simulink model "trail2"  (R2014a)
settings: Solver=ode45  StartTime=0.0  StopTime=10.0  RelTol=1e-3
libraries: simulink x1
settings Model: Creator=Mostafa  LastModifiedBy=Mostafa

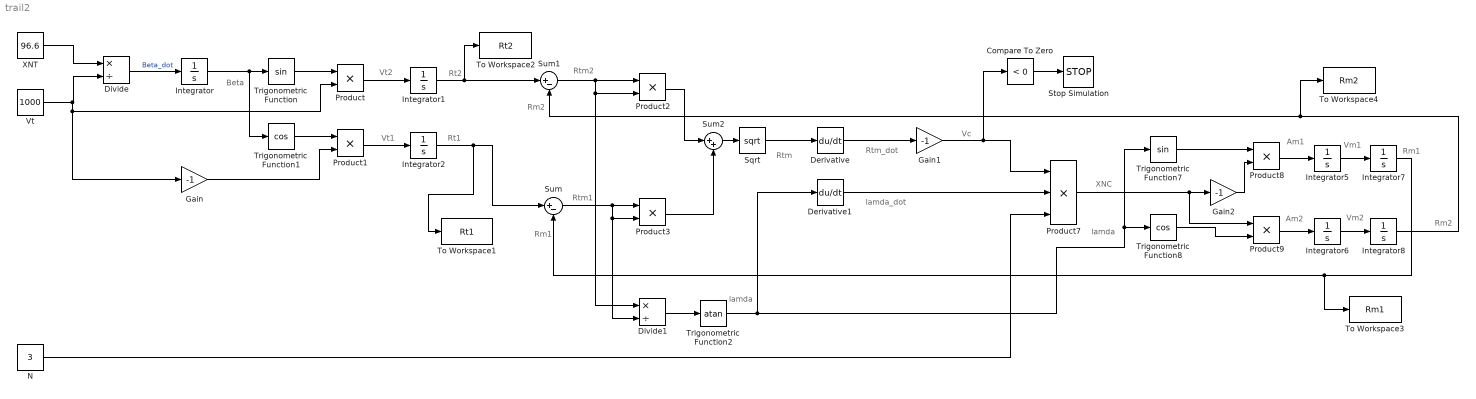
== system trail2 ==
  note: Rm2
  note: Rm1
  note: Vm1
  note: Vm2
  note: Am2
  note: Am1
  note: lamda
  note: XNC
  note: lamda_dot
  note: Vc
  note: Rtm_dot
  note: Rtm
  note: lamda
  note: Rtm2
  note: Rm2
  note: Rtm1
  note: Rm1
  note: Rt1
  note: Rt2
  note: Vt2
  note: Vt1
  note: Beta
  Compare To Zero : simulink/Logic and Bit Operations/Compare To Zero  relop=<  OutDataTypeStr=boolean  ZeroCross=off
  Derivative : Derivative
  Derivative1 : Derivative
  Divide : Product  Inputs=*/
  Divide1 : Product  Inputs=*/
  Gain : Gain  Gain=-1
  Gain1 : Gain  Gain=-1
  Gain2 : Gain  Gain=-1
  Integrator{,5..7} (4 alike) : Integrator
  Integrator1 : Integrator  InitialCondition=10000
  Integrator2 : Integrator  InitialCondition=12000
  Integrator8 : Integrator  InitialCondition=9000
  N : Constant  Value=3
  Product{,1..3,8..9} (6 alike) : Product
  Product7 : Product  Inputs=3
  Sqrt : Sqrt  SaturateOnIntegerOverflow=on
  Stop Simulation : Stop
  Sum : Sum  Inputs=|+-
  Sum1 : Sum  Inputs=|+-
  Sum2 : Sum  Inputs=|++
  To Workspace1 : ToWorkspace  VariableName=Rt1  SampleTime=-1
  To Workspace2 : ToWorkspace  VariableName=Rt2  SampleTime=-1
  To Workspace3 : ToWorkspace  VariableName=Rm1  SampleTime=-1
  To Workspace4 : ToWorkspace  VariableName=Rm2  SampleTime=-1
  Trigonometric Function : Trigonometry
  Trigonometric Function1 : Trigonometry  Operator=cos
  Trigonometric Function2 : Trigonometry  Operator=atan
  Trigonometric Function7 : Trigonometry
  Trigonometric Function8 : Trigonometry  Operator=cos
  "Vt " : Constant  Value=1000
  XNT : Constant  Value=96.6
  wires:
  XNT/1 -> Divide/1
  "Vt "/1 -> Gain/1, Product/2, Divide/2
  Divide/1 -> Integrator/1  "Beta_dot"
  Integrator/1 -> Trigonometric Function1/1, Trigonometric Function/1
  Trigonometric Function/1 -> Product/1
  Gain/1 -> Product1/2
  Trigonometric Function1/1 -> Product1/1
  Product1/1 -> Integrator2/1
  Product/1 -> Integrator1/1
  Integrator1/1 -> To Workspace2/1, Sum1/1
  Integrator2/1 -> To Workspace1/1, Sum/1
  Sum1/1 -> Product2/2, Divide1/1, Product2/1
  Sum/1 -> Divide1/2, Product3/2, Product3/1
  Product2/1 -> Sum2/1
  Product3/1 -> Sum2/2
  Sum2/1 -> Sqrt/1
  Divide1/1 -> Trigonometric Function2/1
  Trigonometric Function2/1 -> Derivative1/1, Trigonometric Function7/1, Trigonometric Function8/1
  Sqrt/1 -> Derivative/1
  Derivative/1 -> Gain1/1
  Gain1/1 -> Compare To Zero/1, Product7/1
  Derivative1/1 -> Product7/2
  N/1 -> Product7/3
  Product7/1 -> Product9/1, Gain2/1
  Trigonometric Function8/1 -> Product9/2
  Gain2/1 -> Product8/2
  Trigonometric Function7/1 -> Product8/1
  Product8/1 -> Integrator5/1
  Product9/1 -> Integrator6/1
  Integrator6/1 -> Integrator8/1
  Integrator5/1 -> Integrator7/1
  Compare To Zero/1 -> Stop Simulation/1
  Integrator7/1 -> To Workspace3/1, Sum/2
  Integrator8/1 -> To Workspace4/1, Sum1/2
